simulink model "Test_Byte_Multiplexer_4_to_1"  (R2023a)
settings: Solver=ode45  StartTime=0.0  StopTime=len  RelTol=1e-3  EnableMultiTasking=on
libraries: Miscellaneous x5, Byte_Multiplexers_Lib x1, simulink x1
settings Model: Creator=N  LastModifiedBy=Jozko Mrkvicka
settings SolverCC: AlgebraicLoopSolver=TrustRegion
settings DataIOCC: SaveFormat=Array  ReturnWorkspaceOutputs=off
settings OptimizationCC: LifeSpan=inf
settings DebuggingCC: UnconnectedInputMsg=warning  UnconnectedOutputMsg=warning  UnconnectedLineMsg=warning  SFUnexpectedBacktrackingDiag=warning  SFNoUnconditionalDefaultTransitionDiag=warning  ArithmeticOperatorsInVariantConditions=warning
settings HardwareCC: ProdWordSize=32
settings ModelReferenceCC: EnableRefExpFcnMdlSchedulingChecks=on
settings SFSimCC: SimUseLocalCustomCode=off  CustomCodeUndefinedFunction=UseInterfaceOnly
settings RTWCC: RTWUseLocalCustomCode=off
settings CodeAppCC: StateflowObjectComments=on
settings GRTTargetCC: TargetLangStandard=C89/C90 (ANSI)
settings ConfigComp: CovMetricSettings=dw  CovSaveCumulativeToWorkspaceVar=on  CovSaveSingleToWorkspaceVar=on  CovExternalEMLEnable=off

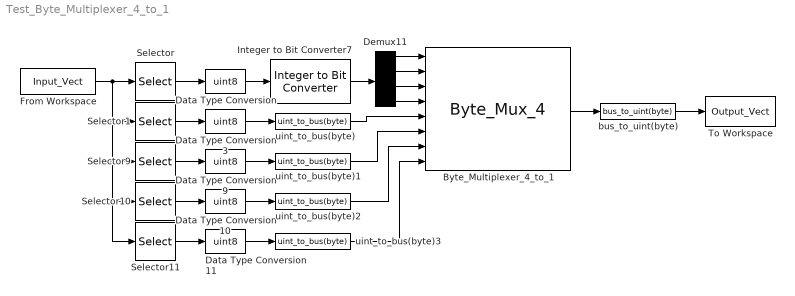
== system Test_Byte_Multiplexer_4_to_1 ==
  Byte_Multiplexer_4_to_1 : Byte_Multiplexers_Lib/Byte_Mux_4  SystemSampleTime=-1  VariantActivationTime=update diagram  Latency=0  AutoFrameSizeCalculation=off
  Data Type Conversion{,3,9..11} (5 alike) : DataTypeConversion  OutDataTypeStr=uint8  SaturateOnIntegerOverflow=off  RndMeth=Floor
  Demux11 : Demux
  From Workspace : FromWorkspace  VariableName=Input_Vect  SampleTime=1  Interpolate=off  ZeroCross=off  OutputAfterFinalValue=Holding final value
  Integer to Bit Converter7 : simulink/Logic and Bit Operations/Integer to Bit Converter  nbits=4  signedInputValues=Unsigned  bitOrder=MSB first  outDtype=boolean
      settings: LibrarySourceBlock=|
      | commutil2/Integer to Bit
      | Converter
  Selector : Selector  IndexMode=Zero-based  InputPortWidth=5  SampleTime=1  IndexOptions=Index vector (dialog)  Indices=0  OutputSizes=1
  Selector1 : Selector  IndexMode=Zero-based  InputPortWidth=5  IndexOptions=Index vector (dialog)  Indices=1  OutputSizes=1
  Selector10 : Selector  IndexMode=Zero-based  InputPortWidth=5  IndexOptions=Index vector (dialog)  Indices=3  OutputSizes=1
  Selector11 : Selector  IndexMode=Zero-based  InputPortWidth=5  IndexOptions=Index vector (dialog)  Indices=4  OutputSizes=1
  Selector9 : Selector  IndexMode=Zero-based  InputPortWidth=5  IndexOptions=Index vector (dialog)  Indices=2  OutputSizes=1
  To Workspace : ToWorkspace  VariableName=Output_Vect  SampleTime=1
  bus_to_uint(byte) : Miscellaneous/bus_to_uint(byte)  SystemSampleTime=-1  VariantActivationTime=update diagram  Latency=0  AutoFrameSizeCalculation=off
  uint_to_bus(byte){,1..3} (4 alike) : Miscellaneous/uint_to_bus(byte)  SystemSampleTime=-1  VariantActivationTime=update diagram  Latency=0  AutoFrameSizeCalculation=off
  wires:
  Byte_Multiplexer_4_to_1/1 -> bus_to_uint(byte)/1
  Demux11/2 -> Byte_Multiplexer_4_to_1/2
  Integer to Bit Converter7/1 -> Demux11/1
  Demux11/1 -> Byte_Multiplexer_4_to_1/1
  Selector/1 -> Data Type Conversion/1
  Selector1/1 -> Data Type Conversion3/1
  Data Type Conversion3/1 -> uint_to_bus(byte)/1
  Data Type Conversion/1 -> Integer to Bit Converter7/1
  Selector9/1 -> Data Type Conversion9/1
  From Workspace/1 -> Selector11/1, Selector10/1, Selector9/1, Selector1/1, Selector/1
  Selector10/1 -> Data Type Conversion10/1
  Selector11/1 -> Data Type Conversion11/1
  Data Type Conversion9/1 -> uint_to_bus(byte)1/1
  Data Type Conversion10/1 -> uint_to_bus(byte)2/1
  Data Type Conversion11/1 -> uint_to_bus(byte)3/1
  uint_to_bus(byte)/1 -> Byte_Multiplexer_4_to_1/5
  uint_to_bus(byte)1/1 -> Byte_Multiplexer_4_to_1/6
  uint_to_bus(byte)2/1 -> Byte_Multiplexer_4_to_1/7
  uint_to_bus(byte)3/1 -> Byte_Multiplexer_4_to_1/8
  bus_to_uint(byte)/1 -> To Workspace/1
  Demux11/3 -> Byte_Multiplexer_4_to_1/3
  Demux11/4 -> Byte_Multiplexer_4_to_1/4
